simulink model "KineMPC"  (R2024b)
settings: Solver=ode8  StartTime=0.0  StopTime=15  FixedStep=Ts_plant  RelTol=1e-3
values from neighbouring files (symbols this model uses):
  D = [SIGMA ... (first row only)    [LinearMPCPrecomputer.m]    (also in param.mat = [10000 0 -10000 0 0 0 0 0 0 0 0 0 ... (1600 elements, 80x20))
  Dm1 = 0.0    (= 0)    [SimParameters.m]    (also in param.mat)
  Dm2 = 0    [SimParameters.m]    (also in param.mat)
  Dm3 = 0    [SimParameters.m]    (also in param.mat)
  DU_MAX = repmat(du_MAX,P,1)    [LinearMPCPrecomputer.m]    (also in param.mat = [100 100 100 100 100 100 100 100 100 100 100 100 ... (20 ele)
  DU_MIN = repmat(du_MIN,P,1)    [LinearMPCPrecomputer.m]    (also in param.mat = [-100 -100 -100 -100 -100 -100 -100 -100 -100 -100 -100 -100)
  Jm1 = 8.61827e-4    (= 0.000861827)    [SimParameters.m]    (also in param.mat)
  Jm2 = 4.6370e-04    (= 0.0004637)    [SimParameters.m]    (also in param.mat)
  Jm3 = 2.4640e-04    (= 0.0002464)    [SimParameters.m]    (also in param.mat)
  Kpp1 = 2.0    (= 2)    [SimParameters.m]    (also in param.mat = 10)
  Kpp2 = 2.0    (= 2)    [SimParameters.m]    (also in param.mat = 10)
  Kpp3 = 2.0    (= 2)    [SimParameters.m]    (also in param.mat = 10)
  Kt1 = 4* 0.070504    (= 0.282016)    [SimParameters.m]    (also in param.mat)
  Kt2 = (0.07354) * (4)    (= 0.29416)    [SimParameters.m]    (also in param.mat)
  Kt3 = (0.0631765) * (4)    (= 0.252706)    [SimParameters.m]    (also in param.mat)
  Kvi1 = (w1*w1*Jm1)/Kt1    (= 7.6398768155)    [SimParameters.m]    (also in param.mat)
  Kvi2 = (w2*w2*Jm2)/Kt2    (= 3.94088251292)    [SimParameters.m]    (also in param.mat)
  Kvi3 = (w3*w3*Jm3)/Kt3    (= 2.43761525251)    [SimParameters.m]    (also in param.mat)
  Kvp1 = (Jm1*w1*zeta1)/Kt1    (= 0.15279753631)    [SimParameters.m]    (also in param.mat)
  Kvp2 = (Jm2*w2*zeta2)/Kt2    (= 0.0788176502584)    [SimParameters.m]    (also in param.mat)
  Kvp3 = (Jm3*w3*zeta3)/Kt3    (= 0.0487523050501)    [SimParameters.m]    (also in param.mat)
  long_cmd = 70002    [param.mat]
  M = size(J0,2)    [LinearMPCPrecomputer.m]    (also in PredictionMatrices.m = dim_B(2); param.mat = 2)
  n = size(J0,2)    [LinearMPCPrecomputer.m]    (also in SimParameters.m = 2; param.mat = 2; solver_test.m = length(f))
  P = 10    [SimParameters.m]    (also in param.mat)
  pos_ref2 = cmd_rad(:,2)    [make_cmd.m]    (also in param.mat = [-3.79261034417e-08 -1.13778310325e-07 -2.2755662065e-07 -3.; ref23.mat = [-3.79261034417e-08 -1.13778310325e-07 -2.2755662065e-07 -3.)
  pos_ref3 = cmd_rad(:,3)    [make_cmd.m]    (also in param.mat = [7.23144185756e-10 2.16943255727e-09 4.33886511453e-09 7.231; ref23.mat = [7.23144185756e-10 2.16943255727e-09 4.33886511453e-09 7.231)
  Q = q1 + q2    [LinearMPCPrecomputer.m]    (also in param.mat = [0 0 0 0 0 0 0 0 0 0 0 0 ... (400 elements, 20x20)])
  Rg2 = 121    [SimParameters.m]    (also in param.mat)
  Rg3 = 121    [SimParameters.m]    (also in param.mat)
  Sa = kron(SSa,eye(M))/(Ts*Ts)    [LinearMPCPrecomputer.m]    (also in param.mat = [100000000 0 -200000000 0 100000000 0 0 0 0 0 0 0 ... (400 e)
  Sv = kron(SSv,eye(M))/Ts    [LinearMPCPrecomputer.m]    (also in param.mat = [10000 0 -10000 0 0 0 0 0 0 0 0 0 ... (400 elements, 20x20)])
  Ts = 100e-6    (= 0.0001)    [SimParameters.m]    (also in make_cmd.m; param.mat)
  Ts_control = 100e-6    (= 0.0001)    [SimParameters.m]    (also in param.mat)
  Ts_MPC = 0.01    [SimParameters.m]    (also in param.mat = 0.0001)
  U_MAX = repmat(u_MAX,P,1)    [LinearMPCPrecomputer.m]    (also in param.mat = [6050 6050 6050 6050 6050 6050 6050 6050 6050 6050 6050 6050)
  U_MIN = repmat(u_MIN,P,1)    [LinearMPCPrecomputer.m]    (also in param.mat = [-6050 -6050 -6050 -6050 -6050 -6050 -6050 -6050 -6050 -6050)
  W_A = eye(n*P)*w_A    [LinearMPCPrecomputer.m]    (also in param.mat = [0 0 0 0 0 0 0 0 0 0 0 0 ... (400 elements, 20x20)])
  W_DU = eye(n*P)*w_DU    [LinearMPCPrecomputer.m]    (also in param.mat = [0 0 0 0 0 0 0 0 0 0 0 0 ... (400 elements, 20x20)])
  W_E = eye(LH*P)*w_E    [LinearMPCPrecomputer.m]    (also in param.mat = [1 0 0 0 0 0 0 0 0 0 0 0 ... (400 elements, 20x20)])
settings Model: Creator=Juan  LastModifiedBy=hi610
settings OptimizationCC: ReuseModelBlockBuffer=off
settings DebuggingCC: UnderSpecifiedDimensionMsg=warning
settings RTWCC: GPUComputeCapability=3.5

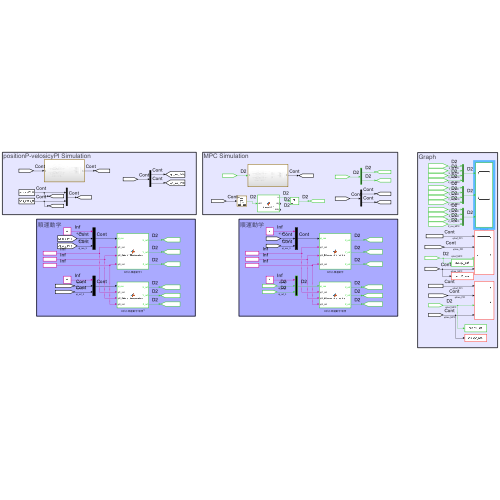
[thumbnail: Simulink's stored preview of the top-level diagram]
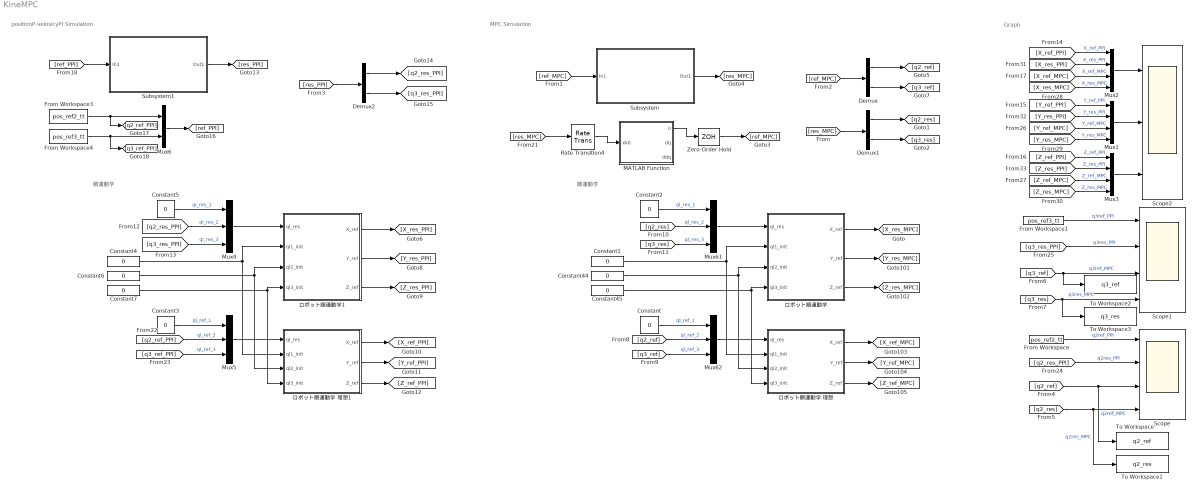
== system KineMPC ==
  note: Graph
  note: MPC Simulation
  note: positionP-velosicyPI Simulation
  note: 順運動学
  note: 順運動学
  Constant{,1..7,44..45} (10 alike) : Constant  Value=0
  Demux : Demux  Outputs=2
  Demux1 : Demux  Outputs=2
  Demux2 : Demux  Outputs=2
  From Workspace : FromWorkspace  VariableName=pos_ref2_tt
  From Workspace1 : FromWorkspace  VariableName=pos_ref3_tt
  From Workspace3 : FromWorkspace  VariableName=pos_ref2_tt
  From Workspace4 : FromWorkspace  VariableName=pos_ref3_tt
  MATLAB Function : MATLAB Function  TreatAsAtomicUnit=on
  Mux1 : Mux
  Mux2 : Mux
  Mux3 : Mux
  Mux{4..5,61..62} (4 alike) : Mux  Inputs=3
  Mux6 : Mux  Inputs=2
  Rate Transition4 : RateTransition  OutPortSampleTime=Ts_MPC
  Scope : Scope  NumInputPorts=4
  Scope1 : Scope  NumInputPorts=4
  Scope2 : Scope  NumInputPorts=3
  Subsystem : Subsystem
  Subsystem1 : Subsystem
  To Workspace : ToWorkspace  VariableName=q2_ref  SaveFormat=Timeseries  SampleTime=-1
  To Workspace1 : ToWorkspace  VariableName=q2_res  SaveFormat=Timeseries  SampleTime=-1
  To Workspace2 : ToWorkspace  VariableName=q3_ref  SaveFormat=Timeseries  SampleTime=-1
  To Workspace3 : ToWorkspace  VariableName=q3_res  SaveFormat=Timeseries  SampleTime=-1
  Zero-Order Hold : ZeroOrderHold  SampleTime=Ts_control
  ロボット順運動学 : MATLAB Function  TreatAsAtomicUnit=on  SystemSampleTime=Ts
  ロボット順運動学 理想 : MATLAB Function  TreatAsAtomicUnit=on  SystemSampleTime=Ts
  ロボット順運動学 理想1 : MATLAB Function  TreatAsAtomicUnit=on  SystemSampleTime=Ts
  ロボット順運動学1 : MATLAB Function  TreatAsAtomicUnit=on  SystemSampleTime=Ts
  wires:
  Rate Transition4/1 -> MATLAB Function/1(xk0)
  Zero-Order Hold/1 -> [ref_MPC]
  Subsystem/1(Out1) -> [res_MPC]
  MATLAB Function/1(u) -> Zero-Order Hold/1
  [ref_MPC] -> Demux/1
  Demux/1 -> [q2_ref]
  Demux/2 -> [q3_ref]
  Demux1/1 -> [q2_res]
  Demux1/2 -> [q3_res]
  [res_MPC] -> Demux1/1
  [res_MPC] -> Rate Transition4/1
  [ref_MPC] -> Subsystem/1(In1)
  [q2_ref] -> To Workspace/1, Scope/3  "q2ref_MPC"
  [q2_res] -> To Workspace1/1, Scope/4  "q2res_MPC"
  [q3_ref] -> To Workspace2/1, Scope1/3  "q3ref_MPC"
  [q3_res] -> Scope1/4, To Workspace3/1  "q3res_MPC"
  From Workspace1/1 -> Scope1/1  "q3ref_PPI"
  [Z_ref_PPI] -> Mux3/1  "Z_ref_PPI"
  [Z_res_MPC] -> Mux3/4  "Z_res_MPC"
  Mux3/1 -> Scope2/3
  Subsystem1/1(Out1) -> [res_PPI]
  [res_PPI] -> Demux2/1
  Demux2/2 -> [q3_res_PPI]
  Demux2/1 -> [q2_res_PPI]
  From Workspace4/1 -> [q3_ref_PPI], Mux6/2
  From Workspace3/1 -> [q2_ref_PPI], Mux6/1
  Mux6/1 -> [ref_PPI]
  [ref_PPI] -> Subsystem1/1(In1)
  ロボット順運動学/3(Z_ref) -> [Z_res_MPC]
  Constant44/1 -> ロボット順運動学 理想/3(ql2_init), ロボット順運動学/3(ql2_init)
  ロボット順運動学/1(X_ref) -> [X_res_MPC]
  Constant1/1 -> ロボット順運動学 理想/2(ql1_init), ロボット順運動学/2(ql1_init)
  [q3_res] -> Mux61/3  "ql_res_3"
  Constant/1 -> Mux62/1  "ql_ref_1"
  Constant45/1 -> ロボット順運動学 理想/4(ql3_init), ロボット順運動学/4(ql3_init)
  [q3_ref] -> Mux62/3  "ql_ref_3"
  ロボット順運動学 理想/3(Z_ref) -> [Z_ref_MPC]
  Mux62/1 -> ロボット順運動学 理想/1(ql_res)
  ロボット順運動学 理想/2(Y_ref) -> [Y_ref_MPC]
  [q2_res] -> Mux61/2  "ql_res_2"
  Constant2/1 -> Mux61/1  "ql_res_1"
  ロボット順運動学 理想/1(X_ref) -> [X_ref_MPC]
  ロボット順運動学/2(Y_ref) -> [Y_res_MPC]
  Mux61/1 -> ロボット順運動学/1(ql_res)
  [q2_ref] -> Mux62/2  "ql_ref_2"
  [q3_ref_PPI] -> Mux5/3  "ql_ref_3"
  [q2_ref_PPI] -> Mux5/2  "ql_ref_2"
  ロボット順運動学1/3(Z_ref) -> [Z_res_PPI]
  Constant5/1 -> Mux4/1  "ql_res_1"
  ロボット順運動学1/2(Y_ref) -> [Y_res_PPI]
  Mux4/1 -> ロボット順運動学1/1(ql_res)
  Constant7/1 -> ロボット順運動学 理想1/4(ql3_init), ロボット順運動学1/4(ql3_init)
  ロボット順運動学 理想1/3(Z_ref) -> [Z_ref_PPI]
  Constant3/1 -> Mux5/1  "ql_ref_1"
  ロボット順運動学 理想1/2(Y_ref) -> [Y_ref_PPI]
  Mux5/1 -> ロボット順運動学 理想1/1(ql_res)
  ロボット順運動学 理想1/1(X_ref) -> [X_ref_PPI]
  [q3_res_PPI] -> Mux4/3  "ql_res_3"
  ロボット順運動学1/1(X_ref) -> [X_res_PPI]
  Constant4/1 -> ロボット順運動学 理想1/2(ql1_init), ロボット順運動学1/2(ql1_init)
  Constant6/1 -> ロボット順運動学 理想1/3(ql2_init), ロボット順運動学1/3(ql2_init)
  [q2_res_PPI] -> Mux4/2  "ql_res_2"
  [q2_res_PPI] -> Scope/2  "q2res_PPI"
  [q3_res_PPI] -> Scope1/2  "q3res_PPI"
  From Workspace/1 -> Scope/1  "q2ref_PPI"
  [Z_ref_MPC] -> Mux3/3  "Z_ref_MPC"
  [Z_res_PPI] -> Mux3/2  "Z_res_PPI"
  [Y_ref_PPI] -> Mux1/1  "Y_ref_PPI"
  [Y_res_PPI] -> Mux1/2  "Y_res_PPI"
  [Y_ref_MPC] -> Mux1/3  "Y_ref_MPC"
  [Y_res_MPC] -> Mux1/4  "Y_res_MPC"
  Mux1/1 -> Scope2/2
  Mux2/1 -> Scope2/1
  [X_res_MPC] -> Mux2/4  "X_res_MPC"
  [X_ref_MPC] -> Mux2/3  "X_ref_MPC"
  [X_res_PPI] -> Mux2/2  "X_res_PPI"
  [X_ref_PPI] -> Mux2/1  "X_ref_PPI"

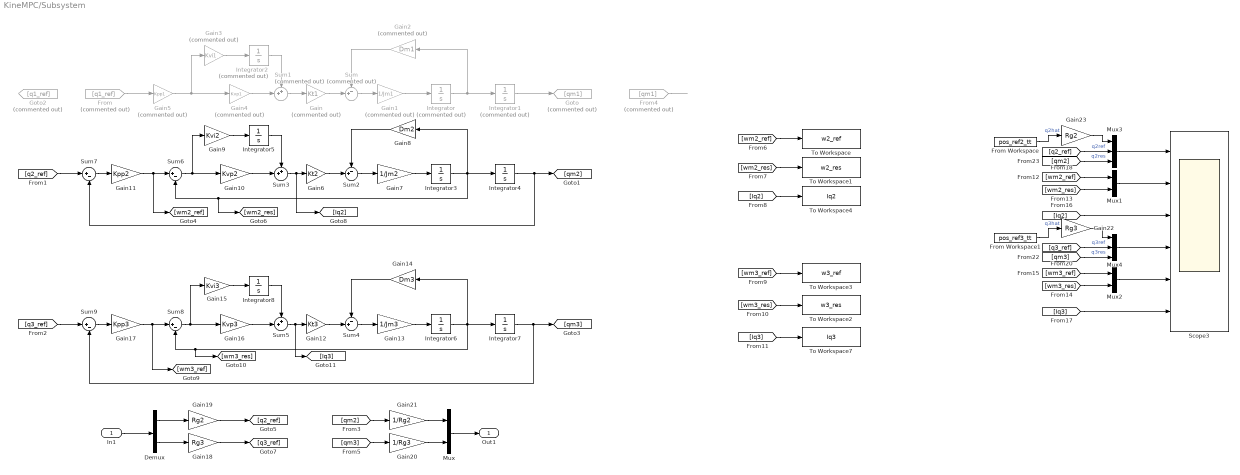
== system KineMPC/Subsystem ==
  In1 : Inport
  Demux : Demux  Outputs=2
  From : From  Commented=on  GotoTag=q1_ref
  From Workspace : FromWorkspace  VariableName=pos_ref2_tt
  From Workspace1 : FromWorkspace  VariableName=pos_ref3_tt
  From4 : From  Commented=on  GotoTag=qm1
  Gain : Gain  Commented=on  Gain=Kt1
  Gain1 : Gain  Commented=on  Gain=1/Jm1
  Gain10 : Gain  Gain=Kvp2
  Gain11 : Gain  Gain=Kpp2
  Gain12 : Gain  Gain=Kt3
  Gain13 : Gain  Gain=1/Jm3
  Gain14 : Gain  Gain=Dm3
  Gain15 : Gain  Gain=Kvi3
  Gain16 : Gain  Gain=Kvp3
  Gain17 : Gain  Gain=Kpp3
  Gain18 : Gain  Gain=Rg3
  Gain19 : Gain  Gain=Rg2
  Gain2 : Gain  Commented=on  Gain=Dm1
  Gain20 : Gain  Gain=1/Rg3
  Gain21 : Gain  Gain=1/Rg2
  Gain22 : Gain  Gain=Rg3
  Gain23 : Gain  Gain=Rg2
  Gain3 : Gain  Commented=on  Gain=Kvi1
  Gain4 : Gain  Commented=on  Gain=Kvp1
  Gain5 : Gain  Commented=on  Gain=Kpp1
  Gain6 : Gain  Gain=Kt2
  Gain7 : Gain  Gain=1/Jm2
  Gain8 : Gain  Gain=Dm2
  Gain9 : Gain  Gain=Kvi2
  Goto : Goto  Commented=on  GotoTag=qm1
  Goto2 : Goto  Commented=on  GotoTag=q1_ref
  Integrator : Integrator  Commented=on
  Integrator1 : Integrator  Commented=on
  Integrator2 : Integrator  Commented=on
  Integrator{3..8} (6 alike) : Integrator
  Mux : Mux  Inputs=2
  Mux1 : Mux  Inputs=2
  Mux2 : Mux  Inputs=2
  Mux3 : Mux  Inputs=3
  Mux4 : Mux  Inputs=3
  Scope3 : Scope  NumInputPorts=6
  Sum : Sum  Commented=on  Inputs=-+|
  Sum1 : Sum  Commented=on  Inputs=++|
  Sum2 : Sum  Inputs=-+|
  Sum3 : Sum  Inputs=++|
  Sum4 : Sum  Inputs=-+|
  Sum5 : Sum  Inputs=++|
  Sum{6..9} (4 alike) : Sum  Inputs=|+-
  To Workspace : ToWorkspace  VariableName=w2_ref  SaveFormat=Timeseries  SampleTime=-1
  To Workspace1 : ToWorkspace  VariableName=w2_res  SaveFormat=Timeseries  SampleTime=-1
  To Workspace2 : ToWorkspace  VariableName=w3_res  SaveFormat=Timeseries  SampleTime=-1
  To Workspace3 : ToWorkspace  VariableName=w3_ref  SaveFormat=Timeseries  SampleTime=-1
  To Workspace4 : ToWorkspace  VariableName=Iq2  SaveFormat=Timeseries  SampleTime=-1
  To Workspace7 : ToWorkspace  VariableName=Iq3  SaveFormat=Timeseries  SampleTime=-1
  Out1 : Outport
  wires:
  Gain1/1 -> Integrator/1
  Integrator/1 -> Gain2/1, Integrator1/1
  Integrator1/1 -> Goto/1
  Sum/1 -> Gain1/1
  In1/1 -> Demux/1
  Demux/1 -> Gain19/1
  Demux/2 -> Gain18/1
  Gain2/1 -> Sum/1
  Gain/1 -> Sum/2
  Sum1/1 -> Gain/1
  Gain3/1 -> Integrator2/1
  Integrator2/1 -> Sum1/1
  Gain4/1 -> Sum1/2
  Gain5/1 -> Gain3/1, Gain4/1
  From/1 -> Gain5/1
  [q2_ref] -> Sum7/1
  Gain10/1 -> Sum3/2
  Integrator5/1 -> Sum3/1
  Gain8/1 -> Sum2/1
  Gain9/1 -> Integrator5/1
  Gain6/1 -> Sum2/2
  Sum2/1 -> Gain7/1
  Integrator4/1 -> Sum7/2, [qm2]
  Gain7/1 -> Integrator3/1
  Sum3/1 -> [Iq2], Gain6/1
  [q3_ref] -> Sum9/1
  Gain16/1 -> Sum5/2
  Integrator8/1 -> Sum5/1
  Gain14/1 -> Sum4/1
  Gain15/1 -> Integrator8/1
  Gain12/1 -> Sum4/2
  Sum4/1 -> Gain13/1
  Integrator7/1 -> [qm3], Sum9/2
  Gain13/1 -> Integrator6/1
  Integrator6/1 -> [wm3_res], Sum8/2, Gain14/1, Integrator7/1
  Sum5/1 -> [Iq3], Gain12/1
  Mux/1 -> Out1/1
  [qm2] -> Gain21/1
  [qm3] -> Gain20/1
  From4/1 -> ?
  Sum7/1 -> Gain11/1
  Gain11/1 -> [wm2_ref], Sum6/1
  Sum6/1 -> Gain9/1, Gain10/1
  Sum9/1 -> Gain17/1
  Sum8/1 -> Gain15/1, Gain16/1
  Integrator3/1 -> [wm2_res], Sum6/2, Gain8/1, Integrator4/1
  Gain17/1 -> [wm3_ref], Sum8/1
  [Iq3] -> To Workspace7/1
  [wm3_res] -> To Workspace2/1
  [wm3_ref] -> To Workspace3/1
  [Iq2] -> To Workspace4/1
  [wm2_res] -> To Workspace1/1
  [wm2_ref] -> To Workspace/1
  Gain18/1 -> [q3_ref]
  Gain19/1 -> [q2_ref]
  Gain20/1 -> Mux/2
  Gain21/1 -> Mux/1
  [wm2_ref] -> Mux1/1
  [wm2_res] -> Mux1/2
  [wm3_ref] -> Mux2/1
  [wm3_res] -> Mux2/2
  Mux2/1 -> Scope3/5
  Mux1/1 -> Scope3/2
  [Iq2] -> Scope3/3
  [Iq3] -> Scope3/6
  Mux3/1 -> Scope3/1
  [qm3] -> Mux4/3  "q3res"
  From Workspace1/1 -> Gain22/1  "q3hat"
  [q3_ref] -> Mux4/2  "q3ref"
  From Workspace/1 -> Gain23/1  "q2hat"
  [q2_ref] -> Mux3/2  "q2ref"
  [qm2] -> Mux3/3  "q2res"
  Mux4/1 -> Scope3/4
  Gain23/1 -> Mux3/1
  Gain22/1 -> Mux4/1

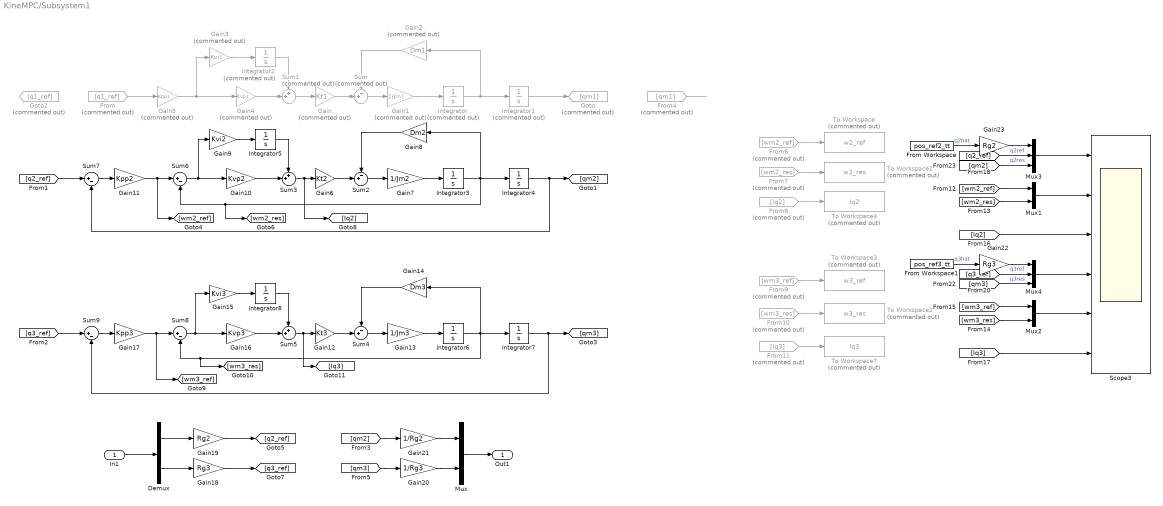
== system KineMPC/Subsystem1 ==
  In1 : Inport
  Demux : Demux  Outputs=2
  From : From  Commented=on  GotoTag=q1_ref
  From Workspace : FromWorkspace  VariableName=pos_ref2_tt
  From Workspace1 : FromWorkspace  VariableName=pos_ref3_tt
  From10 : From  Commented=on  GotoTag=wm3_res
  From11 : From  Commented=on  GotoTag=Iq3
  From4 : From  Commented=on  GotoTag=qm1
  From6 : From  Commented=on  GotoTag=wm2_ref
  From7 : From  Commented=on  GotoTag=wm2_res
  From8 : From  Commented=on  GotoTag=Iq2
  From9 : From  Commented=on  GotoTag=wm3_ref
  Gain : Gain  Commented=on  Gain=Kt1
  Gain1 : Gain  Commented=on  Gain=1/Jm1
  Gain10 : Gain  Gain=Kvp2
  Gain11 : Gain  Gain=Kpp2
  Gain12 : Gain  Gain=Kt3
  Gain13 : Gain  Gain=1/Jm3
  Gain14 : Gain  Gain=Dm3
  Gain15 : Gain  Gain=Kvi3
  Gain16 : Gain  Gain=Kvp3
  Gain17 : Gain  Gain=Kpp3
  Gain18 : Gain  Gain=Rg3
  Gain19 : Gain  Gain=Rg2
  Gain2 : Gain  Commented=on  Gain=Dm1
  Gain20 : Gain  Gain=1/Rg3
  Gain21 : Gain  Gain=1/Rg2
  Gain22 : Gain  Gain=Rg3
  Gain23 : Gain  Gain=Rg2
  Gain3 : Gain  Commented=on  Gain=Kvi1
  Gain4 : Gain  Commented=on  Gain=Kvp1
  Gain5 : Gain  Commented=on  Gain=Kpp1
  Gain6 : Gain  Gain=Kt2
  Gain7 : Gain  Gain=1/Jm2
  Gain8 : Gain  Gain=Dm2
  Gain9 : Gain  Gain=Kvi2
  Goto : Goto  Commented=on  GotoTag=qm1
  Goto2 : Goto  Commented=on  GotoTag=q1_ref
  Integrator : Integrator  Commented=on
  Integrator1 : Integrator  Commented=on
  Integrator2 : Integrator  Commented=on
  Integrator{3..8} (6 alike) : Integrator
  Mux : Mux  Inputs=2
  Mux1 : Mux  Inputs=2
  Mux2 : Mux  Inputs=2
  Mux3 : Mux  Inputs=3
  Mux4 : Mux  Inputs=3
  Scope3 : Scope  NumInputPorts=6
  Sum : Sum  Commented=on  Inputs=-+|
  Sum1 : Sum  Commented=on  Inputs=++|
  Sum2 : Sum  Inputs=-+|
  Sum3 : Sum  Inputs=++|
  Sum4 : Sum  Inputs=-+|
  Sum5 : Sum  Inputs=++|
  Sum{6..9} (4 alike) : Sum  Inputs=|+-
  To Workspace : ToWorkspace  Commented=on  VariableName=w2_ref  SaveFormat=Timeseries  SampleTime=-1
  To Workspace1 : ToWorkspace  Commented=on  VariableName=w2_res  SaveFormat=Timeseries  SampleTime=-1
  To Workspace2 : ToWorkspace  Commented=on  VariableName=w3_res  SaveFormat=Timeseries  SampleTime=-1
  To Workspace3 : ToWorkspace  Commented=on  VariableName=w3_ref  SaveFormat=Timeseries  SampleTime=-1
  To Workspace4 : ToWorkspace  Commented=on  VariableName=Iq2  SaveFormat=Timeseries  SampleTime=-1
  To Workspace7 : ToWorkspace  Commented=on  VariableName=Iq3  SaveFormat=Timeseries  SampleTime=-1
  Out1 : Outport
  wires:
  Gain1/1 -> Integrator/1
  Integrator/1 -> Gain2/1, Integrator1/1
  Integrator1/1 -> Goto/1
  Sum/1 -> Gain1/1
  In1/1 -> Demux/1
  Demux/1 -> Gain19/1
  Demux/2 -> Gain18/1
  Gain2/1 -> Sum/1
  Gain/1 -> Sum/2
  Sum1/1 -> Gain/1
  Gain3/1 -> Integrator2/1
  Integrator2/1 -> Sum1/1
  Gain4/1 -> Sum1/2
  Gain5/1 -> Gain3/1, Gain4/1
  From/1 -> Gain5/1
  [q2_ref] -> Sum7/1
  Gain10/1 -> Sum3/2
  Integrator5/1 -> Sum3/1
  Gain8/1 -> Sum2/1
  Gain9/1 -> Integrator5/1
  Gain6/1 -> Sum2/2
  Sum2/1 -> Gain7/1
  Integrator4/1 -> Sum7/2, [qm2]
  Gain7/1 -> Integrator3/1
  Sum3/1 -> [Iq2], Gain6/1
  [q3_ref] -> Sum9/1
  Gain16/1 -> Sum5/2
  Integrator8/1 -> Sum5/1
  Gain14/1 -> Sum4/1
  Gain15/1 -> Integrator8/1
  Gain12/1 -> Sum4/2
  Sum4/1 -> Gain13/1
  Integrator7/1 -> [qm3], Sum9/2
  Gain13/1 -> Integrator6/1
  Integrator6/1 -> [wm3_res], Sum8/2, Gain14/1, Integrator7/1
  Sum5/1 -> [Iq3], Gain12/1
  Mux/1 -> Out1/1
  [qm2] -> Gain21/1
  [qm3] -> Gain20/1
  From4/1 -> ?
  Sum7/1 -> Gain11/1
  Gain11/1 -> [wm2_ref], Sum6/1
  Sum6/1 -> Gain9/1, Gain10/1
  Sum9/1 -> Gain17/1
  Sum8/1 -> Gain15/1, Gain16/1
  Integrator3/1 -> [wm2_res], Sum6/2, Gain8/1, Integrator4/1
  Gain17/1 -> [wm3_ref], Sum8/1
  From11/1 -> To Workspace7/1
  From10/1 -> To Workspace2/1
  From9/1 -> To Workspace3/1
  From8/1 -> To Workspace4/1
  From7/1 -> To Workspace1/1
  From6/1 -> To Workspace/1
  Gain18/1 -> [q3_ref]
  Gain19/1 -> [q2_ref]
  Gain20/1 -> Mux/2
  Gain21/1 -> Mux/1
  [wm2_ref] -> Mux1/1
  [wm2_res] -> Mux1/2
  [wm3_ref] -> Mux2/1
  [wm3_res] -> Mux2/2
  Mux2/1 -> Scope3/5
  Mux1/1 -> Scope3/2
  [Iq2] -> Scope3/3
  [Iq3] -> Scope3/6
  Mux3/1 -> Scope3/1
  [qm3] -> Mux4/3  "q3res"
  From Workspace1/1 -> Gain22/1  "q3hat"
  [q3_ref] -> Mux4/2  "q3ref"
  From Workspace/1 -> Gain23/1  "q2hat"
  [q2_ref] -> Mux3/2  "q2ref"
  [qm2] -> Mux3/3  "q2res"
  Mux4/1 -> Scope3/4
  Gain23/1 -> Mux3/1
  Gain22/1 -> Mux4/1

== matlab function KineMPC/ロボット順運動学1 ==
  data: ql_res input size=3; ql1_init input; X_ref output size=1; Y_ref output size=1; Z_ref output size=1; ql2_init input; ql3_init input

function [X_ref, Y_ref, Z_ref] = FowardKinematiics(ql_res, ql1_init, ql2_init, ql3_init)
%% 軸角度
q1 = ql1_init + ql_res(1);
q2 = ql2_init + ql_res(2);
q3 = ql3_init + ql_res(3);
q4 = 0;
q5 = 0;
q6 = 0;
    
%% パラメータ
% 各関節角度(rad)
theta1 = q1;
theta2 = -q2;
theta3 = q3;
theta4 = q4;
theta5 = q5;
theta6 = q6;

%　各リンクの長さ
Lac = 0.2685;
Lb  = 0.16;
Ld  = 0.0880;
Le  = 0.56;
Lf  = 0.088;
Lg  = 0.13;
Lh1 = 0.145;
Lh2 = 0.455;
Lii = 0.04;
Lj  = 0.2;
Lk  = 0.05;

% 各関節の座標系から見て次の関節がどこにあるか
p01 = [0;0;0]; %絶対座標と原点が同じ
p12 = [Lb; 0; Lac];
p23 = [ 0; -Ld; Le];
p34 = [ Lh1; Lf; Lg];
p45 = [ Lh2; 0; 0];
p56 = [ Lj; 0; Lii];
p6 = [ Lk; 0; 0];

R1 = [ cos(theta1), -sin(theta1),          0;
       sin(theta1),  cos(theta1),          0;
       0,                0,                1; ];
R2 = [ cos(theta2),         0,   sin(theta2);
       0,                   1,             0;
      -sin(theta2),         0,   cos(theta2); ];
R3 = [ cos(theta3),         0,   sin(theta3);
       0,                   1,             0;
      -sin(theta3),         0,   cos(theta3); ];
R4 = [ 1,                0,                 0;
       0,          cos(theta4),  -sin(theta4);
       0,          sin(theta4),   cos(theta4); ];
R5 = [ cos(theta5),         0,   sin(theta5);
       0,                   1,             0;
      -sin(theta5),         0,   cos(theta5); ];
R6 = [ 1,                0,                 0;
       0,          cos(theta6),  -sin(theta6);
       0,          sin(theta6),   cos(theta6); ];
   

% 回転行列　''は回転軸方向
% R1 = rot('z',theta1);
% R2 = rot('y',theta2);
% R3 = rot('y',theta3);
% R4 = rot('x',theta4);
% R5 = rot('y',theta5);
% R6 = rot('x',theta6);
% R7（先端）は回転なしで長さのみなので省略

%% 手先位置・各関節位置 計算

E = eye(3);
zero = [0, 0, 0];

%　同次変換行列
% 0から1
T01 = [R1,p01;zero,1];
% 1から2
T12 = [R2,p12;zero,1];
% 2から3
T23 = [R3,p23;zero,1];
% 3から4
T34 = [R4,p34;zero,1];
% 4から5
T45 = [R5,p45;zero,1];
% 5から6
T56 = [R6,p56;zero,1];
%6から手先
T6h = [E,p6;zero,1];

%基準座標から各関節までの同次変換行列
T02 = T01*T12;
T03 = T01*T12*T23;
T04 = T01*T12*T23*T34;
T05 = T01*T12*T23*T34*T45;
T06 = T01*T12*T23*T34*T45*T56;
T0h = T01*T12*T23*T34*T45*T56*T6h;

%各関節位置　
r1 = T01(1:3, 4:4);
r2 = T02(1:3, 4:4);
r3 = T03(1:3, 4:4);
r4 = T04(1:3, 4:4);
r5 = T05(1:3, 4:4);
r6 = T06(1:3, 4:4);
rh = T0h(1:3, 4:4);

% グラフ描画用仮想関節(折れ曲がってるとこ)
sub_p12   = [0;0;Lac];
sub_p23   = [0;-Ld;0];
sub_p34_1 = [0;Lf;0];
sub_p34_2 = [0;Lf;Lg];
sub_p56   = [0;0;Lii]; 



r1_sub = T01*[sub_p12;1];
r2_sub = T02*[sub_p23;1];
r3_sub1 = T03*[sub_p34_1;1];
r3_sub2 = T03*[sub_p34_2;1];
r5_sub = T05*[sub_p56;1];

r1_sub = r1_sub(1:3, 1:1);
r2_sub = r2_sub(1:3, 1:1);
r3_sub1 = r3_sub1(1:3, 1:1);
r3_sub2 = r3_sub2(1:3, 1:1);
r5_sub = r5_sub(1:3, 1:1);



%関節位置行列
r = [r1,r2,r3,r4,r5,r6,rh];
r = [r1.';r2.';r3.';r4.';r5.';r6.';rh.'];
%描画用位置行列
r_all = [r1.'; r1_sub.'; r2.'; r2_sub.'; r3.'; r3_sub1.'; r3_sub2.'; r4.'; r5.'; r5_sub.'; r6.'; rh.'];

X_ref = r(7,1);
Y_ref = r(7,2);
Z_ref = r(7,3);

== matlab function KineMPC/ロボット順運動学 ==
  data: ql_res input size=3; ql1_init input; X_ref output size=1; Y_ref output size=1; Z_ref output size=1; ql2_init input; ql3_init input

function [X_ref, Y_ref, Z_ref] = FowardKinematiics(ql_res, ql1_init, ql2_init, ql3_init)
%% 軸角度
q1 = ql1_init + ql_res(1);
q2 = ql2_init + ql_res(2);
q3 = ql3_init + ql_res(3);
q4 = 0;
q5 = 0;
q6 = 0;
    
%% パラメータ
% 各関節角度(rad)
theta1 = q1;
theta2 = -q2;
theta3 = q3;
theta4 = q4;
theta5 = q5;
theta6 = q6;

%　各リンクの長さ
Lac = 0.2685;
Lb  = 0.16;
Ld  = 0.0880;
Le  = 0.56;
Lf  = 0.088;
Lg  = 0.13;
Lh1 = 0.145;
Lh2 = 0.455;
Lii = 0.04;
Lj  = 0.2;
Lk  = 0.05;

% 各関節の座標系から見て次の関節がどこにあるか
p01 = [0;0;0]; %絶対座標と原点が同じ
p12 = [Lb; 0; Lac];
p23 = [ 0; -Ld; Le];
p34 = [ Lh1; Lf; Lg];
p45 = [ Lh2; 0; 0];
p56 = [ Lj; 0; Lii];
p6 = [ Lk; 0; 0];

R1 = [ cos(theta1), -sin(theta1),          0;
       sin(theta1),  cos(theta1),          0;
       0,                0,                1; ];
R2 = [ cos(theta2),         0,   sin(theta2);
       0,                   1,             0;
      -sin(theta2),         0,   cos(theta2); ];
R3 = [ cos(theta3),         0,   sin(theta3);
       0,                   1,             0;
      -sin(theta3),         0,   cos(theta3); ];
R4 = [ 1,                0,                 0;
       0,          cos(theta4),  -sin(theta4);
       0,          sin(theta4),   cos(theta4); ];
R5 = [ cos(theta5),         0,   sin(theta5);
       0,                   1,             0;
      -sin(theta5),         0,   cos(theta5); ];
R6 = [ 1,                0,                 0;
       0,          cos(theta6),  -sin(theta6);
       0,          sin(theta6),   cos(theta6); ];
   

% 回転行列　''は回転軸方向
% R1 = rot('z',theta1);
% R2 = rot('y',theta2);
% R3 = rot('y',theta3);
% R4 = rot('x',theta4);
% R5 = rot('y',theta5);
% R6 = rot('x',theta6);
% R7（先端）は回転なしで長さのみなので省略

%% 手先位置・各関節位置 計算

E = eye(3);
zero = [0, 0, 0];

%　同次変換行列
% 0から1
T01 = [R1,p01;zero,1];
% 1から2
T12 = [R2,p12;zero,1];
% 2から3
T23 = [R3,p23;zero,1];
% 3から4
T34 = [R4,p34;zero,1];
% 4から5
T45 = [R5,p45;zero,1];
% 5から6
T56 = [R6,p56;zero,1];
%6から手先
T6h = [E,p6;zero,1];

%基準座標から各関節までの同次変換行列
T02 = T01*T12;
T03 = T01*T12*T23;
T04 = T01*T12*T23*T34;
T05 = T01*T12*T23*T34*T45;
T06 = T01*T12*T23*T34*T45*T56;
T0h = T01*T12*T23*T34*T45*T56*T6h;

%各関節位置　
r1 = T01(1:3, 4:4);
r2 = T02(1:3, 4:4);
r3 = T03(1:3, 4:4);
r4 = T04(1:3, 4:4);
r5 = T05(1:3, 4:4);
r6 = T06(1:3, 4:4);
rh = T0h(1:3, 4:4);

% グラフ描画用仮想関節(折れ曲がってるとこ)
sub_p12   = [0;0;Lac];
sub_p23   = [0;-Ld;0];
sub_p34_1 = [0;Lf;0];
sub_p34_2 = [0;Lf;Lg];
sub_p56   = [0;0;Lii]; 



r1_sub = T01*[sub_p12;1];
r2_sub = T02*[sub_p23;1];
r3_sub1 = T03*[sub_p34_1;1];
r3_sub2 = T03*[sub_p34_2;1];
r5_sub = T05*[sub_p56;1];

r1_sub = r1_sub(1:3, 1:1);
r2_sub = r2_sub(1:3, 1:1);
r3_sub1 = r3_sub1(1:3, 1:1);
r3_sub2 = r3_sub2(1:3, 1:1);
r5_sub = r5_sub(1:3, 1:1);



%関節位置行列
r = [r1,r2,r3,r4,r5,r6,rh];
r = [r1.';r2.';r3.';r4.';r5.';r6.';rh.'];
%描画用位置行列
r_all = [r1.'; r1_sub.'; r2.'; r2_sub.'; r3.'; r3_sub1.'; r3_sub2.'; r4.'; r5.'; r5_sub.'; r6.'; rh.'];

X_ref = r(7,1);
Y_ref = r(7,2);
Z_ref = r(7,3);

== matlab function KineMPC/ロボット順運動学 理想 ==
  data: ql_res input size=3; ql1_init input; X_ref output size=1; Y_ref output size=1; Z_ref output size=1; ql2_init input size=1; ql3_init input size=1

function [X_ref, Y_ref, Z_ref] = FowardKinematiics(ql_res, ql1_init, ql2_init, ql3_init)
%% 軸角度
q1 = ql1_init + ql_res(1);
q2 = ql2_init + ql_res(2);
q3 = ql3_init + ql_res(3);
q4 = 0;
q5 = 0;
q6 = 0;
    
%% パラメータ
% 各関節角度(deg)
theta1 = q1;
theta2 = -q2;
theta3 = q3;
theta4 = q4;
theta5 = q5;
theta6 = q6;

%　各リンクの長さ
Lac = 0.2685;
Lb  = 0.16;
Ld  = 0.0880;
Le  = 0.56;
Lf  = 0.088;
Lg  = 0.13;
Lh1 = 0.145;
Lh2 = 0.455;
Lii = 0.04;
Lj  = 0.2;
Lk  = 0.05;

% 各関節の座標系から見て次の関節がどこにあるか
p01 = [0;0;0]; %絶対座標と原点が同じ
p12 = [Lb; 0; Lac];
p23 = [ 0; -Ld; Le];
p34 = [ Lh1; Lf; Lg];
p45 = [ Lh2; 0; 0];
p56 = [ Lj; 0; Lii];
p6 = [ Lk; 0; 0];

R1 = [ cos(theta1), -sin(theta1),          0;
       sin(theta1),  cos(theta1),          0;
       0,                0,                1; ];
R2 = [ cos(theta2),         0,   sin(theta2);
       0,                   1,             0;
      -sin(theta2),         0,   cos(theta2); ];
R3 = [ cos(theta3),         0,   sin(theta3);
       0,                   1,             0;
      -sin(theta3),         0,   cos(theta3); ];
R4 = [ 1,                0,                 0;
       0,          cos(theta4),  -sin(theta4);
       0,          sin(theta4),   cos(theta4); ];
R5 = [ cos(theta5),         0,   sin(theta5);
       0,                   1,             0;
      -sin(theta5),         0,   cos(theta5); ];
R6 = [ 1,                0,                 0;
       0,          cos(theta6),  -sin(theta6);
       0,          sin(theta6),   cos(theta6); ];
   

% 回転行列　''は回転軸方向
% R1 = rot('z',theta1);
% R2 = rot('y',theta2);
% R3 = rot('y',theta3);
% R4 = rot('x',theta4);
% R5 = rot('y',theta5);
% R6 = rot('x',theta6);
% R7（先端）は回転なしで長さのみなので省略

%% 手先位置・各関節位置 計算

E = eye(3);
zero = [0, 0, 0];

%　同次変換行列
% 0から1
T01 = [R1,p01;zero,1];
% 1から2
T12 = [R2,p12;zero,1];
% 2から3
T23 = [R3,p23;zero,1];
% 3から4
T34 = [R4,p34;zero,1];
% 4から5
T45 = [R5,p45;zero,1];
% 5から6
T56 = [R6,p56;zero,1];
%6から手先
T6h = [E,p6;zero,1];

%基準座標から各関節までの同次変換行列
T02 = T01*T12;
T03 = T01*T12*T23;
T04 = T01*T12*T23*T34;
T05 = T01*T12*T23*T34*T45;
T06 = T01*T12*T23*T34*T45*T56;
T0h = T01*T12*T23*T34*T45*T56*T6h;

%各関節位置　
r1 = T01(1:3, 4:4);
r2 = T02(1:3, 4:4);
r3 = T03(1:3, 4:4);
r4 = T04(1:3, 4:4);
r5 = T05(1:3, 4:4);
r6 = T06(1:3, 4:4);
rh = T0h(1:3, 4:4);

% グラフ描画用仮想関節(折れ曲がってるとこ)
sub_p12   = [0;0;Lac];
sub_p23   = [0;-Ld;0];
sub_p34_1 = [0;Lf;0];
sub_p34_2 = [0;Lf;Lg];
sub_p56   = [0;0;Lii]; 



r1_sub = T01*[sub_p12;1];
r2_sub = T02*[sub_p23;1];
r3_sub1 = T03*[sub_p34_1;1];
r3_sub2 = T03*[sub_p34_2;1];
r5_sub = T05*[sub_p56;1];

r1_sub = r1_sub(1:3, 1:1);
r2_sub = r2_sub(1:3, 1:1);
r3_sub1 = r3_sub1(1:3, 1:1);
r3_sub2 = r3_sub2(1:3, 1:1);
r5_sub = r5_sub(1:3, 1:1);



%関節位置行列
r = [r1,r2,r3,r4,r5,r6,rh];
r = [r1.';r2.';r3.';r4.';r5.';r6.';rh.'];
%描画用位置行列
r_all = [r1.'; r1_sub.'; r2.'; r2_sub.'; r3.'; r3_sub1.'; r3_sub2.'; r4.'; r5.'; r5_sub.'; r6.'; rh.'];

X_ref = r(7,1);
Y_ref = r(7,2);
Z_ref = r(7,3);

== matlab function KineMPC/ロボット順運動学 理想1 ==
  data: ql_res input size=3; ql1_init input; X_ref output size=1; Y_ref output size=1; Z_ref output size=1; ql2_init input size=1; ql3_init input size=1

function [X_ref, Y_ref, Z_ref] = FowardKinematiics(ql_res, ql1_init, ql2_init, ql3_init)
%% 軸角度
q1 = ql1_init + ql_res(1);
q2 = ql2_init + ql_res(2);
q3 = ql3_init + ql_res(3);
q4 = 0;
q5 = 0;
q6 = 0;
    
%% パラメータ
% 各関節角度(deg)
theta1 = q1;
theta2 = -q2;
theta3 = q3;
theta4 = q4;
theta5 = q5;
theta6 = q6;

%　各リンクの長さ
Lac = 0.2685;
Lb  = 0.16;
Ld  = 0.0880;
Le  = 0.56;
Lf  = 0.088;
Lg  = 0.13;
Lh1 = 0.145;
Lh2 = 0.455;
Lii = 0.04;
Lj  = 0.2;
Lk  = 0.05;

% 各関節の座標系から見て次の関節がどこにあるか
p01 = [0;0;0]; %絶対座標と原点が同じ
p12 = [Lb; 0; Lac];
p23 = [ 0; -Ld; Le];
p34 = [ Lh1; Lf; Lg];
p45 = [ Lh2; 0; 0];
p56 = [ Lj; 0; Lii];
p6 = [ Lk; 0; 0];

R1 = [ cos(theta1), -sin(theta1),          0;
       sin(theta1),  cos(theta1),          0;
       0,                0,                1; ];
R2 = [ cos(theta2),         0,   sin(theta2);
       0,                   1,             0;
      -sin(theta2),         0,   cos(theta2); ];
R3 = [ cos(theta3),         0,   sin(theta3);
       0,                   1,             0;
      -sin(theta3),         0,   cos(theta3); ];
R4 = [ 1,                0,                 0;
       0,          cos(theta4),  -sin(theta4);
       0,          sin(theta4),   cos(theta4); ];
R5 = [ cos(theta5),         0,   sin(theta5);
       0,                   1,             0;
      -sin(theta5),         0,   cos(theta5); ];
R6 = [ 1,                0,                 0;
       0,          cos(theta6),  -sin(theta6);
       0,          sin(theta6),   cos(theta6); ];
   

% 回転行列　''は回転軸方向
% R1 = rot('z',theta1);
% R2 = rot('y',theta2);
% R3 = rot('y',theta3);
% R4 = rot('x',theta4);
% R5 = rot('y',theta5);
% R6 = rot('x',theta6);
% R7（先端）は回転なしで長さのみなので省略

%% 手先位置・各関節位置 計算

E = eye(3);
zero = [0, 0, 0];

%　同次変換行列
% 0から1
T01 = [R1,p01;zero,1];
% 1から2
T12 = [R2,p12;zero,1];
% 2から3
T23 = [R3,p23;zero,1];
% 3から4
T34 = [R4,p34;zero,1];
% 4から5
T45 = [R5,p45;zero,1];
% 5から6
T56 = [R6,p56;zero,1];
%6から手先
T6h = [E,p6;zero,1];

%基準座標から各関節までの同次変換行列
T02 = T01*T12;
T03 = T01*T12*T23;
T04 = T01*T12*T23*T34;
T05 = T01*T12*T23*T34*T45;
T06 = T01*T12*T23*T34*T45*T56;
T0h = T01*T12*T23*T34*T45*T56*T6h;

%各関節位置　
r1 = T01(1:3, 4:4);
r2 = T02(1:3, 4:4);
r3 = T03(1:3, 4:4);
r4 = T04(1:3, 4:4);
r5 = T05(1:3, 4:4);
r6 = T06(1:3, 4:4);
rh = T0h(1:3, 4:4);

% グラフ描画用仮想関節(折れ曲がってるとこ)
sub_p12   = [0;0;Lac];
sub_p23   = [0;-Ld;0];
sub_p34_1 = [0;Lf;0];
sub_p34_2 = [0;Lf;Lg];
sub_p56   = [0;0;Lii]; 



r1_sub = T01*[sub_p12;1];
r2_sub = T02*[sub_p23;1];
r3_sub1 = T03*[sub_p34_1;1];
r3_sub2 = T03*[sub_p34_2;1];
r5_sub = T05*[sub_p56;1];

r1_sub = r1_sub(1:3, 1:1);
r2_sub = r2_sub(1:3, 1:1);
r3_sub1 = r3_sub1(1:3, 1:1);
r3_sub2 = r3_sub2(1:3, 1:1);
r5_sub = r5_sub(1:3, 1:1);



%関節位置行列
r = [r1,r2,r3,r4,r5,r6,rh];
r = [r1.';r2.';r3.';r4.';r5.';r6.';rh.'];
%描画用位置行列
r_all = [r1.'; r1_sub.'; r2.'; r2_sub.'; r3.'; r3_sub1.'; r3_sub2.'; r4.'; r5.'; r5_sub.'; r6.'; rh.'];

X_ref = r(7,1);
Y_ref = r(7,2);
Z_ref = r(7,3);

== matlab function KineMPC/MATLAB Function ==
  data: u output size=2; xk0 input; pos_ref2 parameter; M parameter; Sv parameter; Sa parameter; W_E parameter; W_DU parameter; W_A parameter; Q parameter; D parameter; DU_MAX parameter; DU_MIN parameter; U_MAX parameter; U_MIN parameter; P parameter; n parameter; Ts_MPC parameter; pos_ref3 parameter; long_cmd parameter; dq output; ddq output
function [u,dq,ddq] = LinearMPC(xk0, pos_ref2, M, Sv, Sa, W_E, W_DU, W_A, Q, D, DU_MAX, DU_MIN, U_MAX, U_MIN, P, n, Ts_MPC, pos_ref3, long_cmd)
%{
LinearMPC for Simulink

Solve the following quadratic program for every sample:

min  0.5*z'*H*z + f'*z
z
    s.t.  Dz<=b

where z = [Up | epsilon]' = [u{k} u{k+2} u{k+3} ... u{k+l-1} epsilon]'


***Required parameters (Detailed explanation given below):
For cost function: [H, R1, R2, R3]
For inequality constraints: [D, DU_MAX, DU_MIN, X_MAX, X_MIN, U_MAX, U_MIN, AAbar]
For both: [P, M, LT, L]
(P: Prediction horizon, L: Control horizon, LT: Number of constrained states, M: Input dimension) 
(Use LinearMPCPrecomputer function to compute)


***Input arguments:
-xk0: Last sample state vector X
-uk0: Last sample input vector u
-y_ref: Reference

***Output:
-Up: Computed optimal input vector over prediction horizon
-epsilon: Slack variable value
-x_predic: Predicted state vector over prediction horizon

NOTE: Some matrices need to be multiplied either with xk0 or uk0 to form
the whole quadratic program to be solved, so the precomputed required
parameters are given as below:
%}
% M = 2;
persistent k;
persistent uk0;
persistent duk0;
if isempty(k)
    k = 1;
end
if k > (long_cmd-P+1)
    k = long_cmd-P+1;
end
if isempty(uk0)
    uk0 = zeros(M,1);
end
if isempty(duk0)
    duk0 = zeros(M,1);
end
qref2 = zeros(P,1);
qref3 = zeros(P,1);
qref2(:,1) = pos_ref2(k:k+P-1,1);
qref3(:,1) = pos_ref3(k:k+P-1,1);

%Reference and previous value generation
% qref_P = repmat(qref,P,1);
qref_P = zeros(M*P,1);
Jhat = zeros(M,M,P);
% Jhat_P = kron(eye(P),Jhat);
for c= 1:P
    qref_P(2*(c-1)+1,1) = qref2(c);
    qref_P(2*(c-1)+2,1) = qref3(c);

    % q1,2,3はradで与える
    q2 = qref2(c);
    q3 = qref3(c);
    
    % リンク長
    Le  = 0.56;
    Lg  = 0.13;
    Lh1 = 0.145;
    Lh2 = 0.455;
    Lii = 0.04;
    Lj  = 0.2;
    Lk  = 0.05;
    
    L2 = Le;
    L3 = Lg + Lii;
    L4 = Lh1 + Lh2 + Lj + Lk;
    
    % q1,2,3はdegで与える。ここでradに変換。
    % theta2 = q2 / 180 * pi;
    % theta3 = q3 / 180 * pi;
    theta2 = q2;
    theta3 = q3;
    
    % 三角関数
    S2 = sin(theta2);
    C2 = cos(theta2);
    S23 = sin(theta2 + theta3);
    C23 = cos(theta2 + theta3);
    
    % 各要素の偏微分
    % dxdthe1 = -S1*(L1 + L2*S2 + L3*S23 + L4*C23);
    dxdthe2 = (L2*C2 + L3*C23 - L4*S23);
    dxdthe3 = (L3*C23 - L4*S23);
    % dydthe1 = C1*(L1 + L2*S2 + L3*S23 + L4*C23);
    % dydthe2 = S1*(L2*C2 - L3*C23 - L4*S23);
    % dydthe3 = S1*(L3*C23 - L4*S23);
    % dzdthe1 = 0;
    dzdthe2 = -L2*S2 - L3*S23 - L4*C23;
    dzdthe3 = -L3*S23 - L4*C23;
    
    Jhat(:,:,c) = [dxdthe2 dxdthe3;
                   dzdthe2 dzdthe3];
end
Jhat_P = blkdiag(Jhat(:,:,1),Jhat(:,:,2),Jhat(:,:,3),Jhat(:,:,4),Jhat(:,:,5),Jhat(:,:,6),Jhat(:,:,7),Jhat(:,:,8),Jhat(:,:,9),Jhat(:,:,10));
v = zeros(M*P,1);
v(1:M,:) = -uk0;
v = v/Ts_MPC;
a = zeros(M*P,1);
a(1:M,:) = -uk0-duk0;
a(M+1:2*M,:) = uk0;
a = a/(Ts_MPC*Ts_MPC);

%Cost function 1\2 * H'*z*H + f'*z
%H is already precomputed
%z = [Up | epsilon]^T , where Up-> R(MP x MP), epsilon-> R(1x1)
H = 2*(Jhat_P'*W_E*Jhat_P + Q);
f = 2*(v'*W_DU*Sv + a'*W_A*Sa - qref_P'*Jhat_P'*W_E*Jhat_P)';

%Constraints
%   D*z<=b     (inequality constraints)
%D is already precomputed, b needs to be computed
%Inequalities: [D, DU_MAX, DU_MIN, U_MAX, U_MIN] needs to be precomputed

BMAX_Q = U_MAX;
BMIN_Q = U_MIN;
BMAX_DQ = DU_MAX - v;
BMIN_DQ = DU_MIN - v;
BMAX = [BMAX_DQ;
        BMAX_Q;
        ];    
    
BMIN = [BMIN_DQ;
        BMIN_Q;        
        ];

b = [BMAX;
    -BMIN];

%Solve quadratic program
%{
min  0.5*z'*H*z + f'*z
z
    s.t.  Dz<=b

where z = [Up | epsilon]' = [u{k} u{k+2} u{k+3} ... u{k+L-1} epsilon]'
%}
N = n*P;
opt = mpcInteriorPointOptions;
opt.IntegrityChecks = true;
x0 = zeros(N,1); %Cold start
Deq = zeros(0,N);
beq = zeros(0,1);
% z = [1 1 1 1]';
[z,exitflag] = mpcInteriorPointSolver(H,f,D,b,Deq,beq,x0,opt);
u = z(1:2,1);
dq_full = Sv * z + v;
ddq_full = Sa * z + a;
dq = dq_full;
ddq = ddq_full;
%ufull = zeros(M*P,1);
%ufull = z;

% u = [0; 0];
uk0 = u;
k = k+1;

end
